simulink model "TV_2017old"  (R2016a)
settings: Solver=FixedStepAuto  StartTime=0.0  StopTime=inf  FixedStep=0.001  RelTol=1e-3
PreLoadFcn:
  | TV_2017_parameters
values from neighbouring files (symbols this model uses):
  battery_voltage = single(530)    [HIL_parameters.m]    (also in HIL_parameters_2018.m; TV_2017_parameters.m; TV_2017_parameters_VD.m)
  car_params = Simulink_Car_params    [HIL_parameters.m]    (also in HIL_parameters_2018.m; TV_2017_parameters.m; TV_2017_parameters_VD.m)
  i_Diff = 16    [HIL_parameters.m]    (also in HIL_parameters_2018.m; TV_2017_parameters.m)
  Kp = 1    [HIL_parameters.m]    (also in HIL_parameters_2018.m; TV_2017_parameters.m; TV_2017_parameters_VD.m)
  motor_data = struct    [HIL_parameters.m]    (also in HIL_parameters_2018.m; TV_2017_parameters.m)
  powerLimitControl = Simulink_el    [HIL_parameters.m]    (also in HIL_parameters_2018.m; TV_2017_parameters.m; TV_2017_parameters_VD.m)
  settings = Simulink_Settings    [HIL_parameters.m]    (also in HIL_parameters_2018.m; TV_2017_parameters.m; TV_2017_parameters_VD.m)
  SpdC_BCC = 0    [HIL_parameters.m]    (also in HIL_parameters_2018.m; TV_2017_parameters.m; TV_2017_parameters_VD.m)
  Speed_Neg_sat = -21    [HIL_parameters.m]    (also in HIL_parameters_2018.m; TV_2017_parameters.m; TV_2017_parameters_VD.m)
  Speed_Pos_sat = 21    [HIL_parameters.m]    (also in HIL_parameters_2018.m; TV_2017_parameters.m; TV_2017_parameters_VD.m)
  SteeringAngleFL = [-23.80 -22.65 -21.50 -20.34 -19.18 -18.03 -16.86 -15.70 -14.53 -13.35 -12.18 -10.99 -9.80 -8.61 -7.40 -6.19 -4.97 -3.75 -2.51 -1.26 0 1.27 2.56 3.85 5.17 6.50 7.84 9.21 10.59 12.00 13.42 14.88 16.36 17.87 19.41 20.99 22.61 24.26 25.97 27.73 29.54]    [CarSetupAnalysis2018.m]    (also in HIL_parameters_2018.m; TV_2017_parameters.m; TV_2017_parameters_VD.m = [-24.129 -22.950 -21.772 -20.593 -19.413 -18.232 -17.050 -15)
  SteeringAngleFR = [-29.54 -27.73 -25.97 -24.26 -22.61 -20.99 -19.41 -17.87 -16.36 -14.88 -13.42 -12.00 -10.59 -9.21 -7.84 -6.50 -5.17 -3.85 -2.56 -1.27 0 1.26 2.51 3.75 4.97 6.19 7.40 8.61 9.80 10.99 12.18 13.35 14.53 15.70 16.86 18.03 19.18 20.34 21.50 22.65 23.80]    [CarSetupAnalysis2018.m]    (also in HIL_parameters_2018.m; TV_2017_parameters.m; TV_2017_parameters_VD.m = [-29.3050 -27.5340 -25.8140 -24.1410 -22.5110 -20.9180 -19.3)
  SteeringWhAngle = [-105 -99.75 -94.5 -89.25 -84 -78.75 -73.5 -68.25 -63 -57.75 -52.5 -47.25 -42 -36.75 -31.5 -26.25 -21.0 -15.75 -10.5 -5.25 0.0 5.25 10.50 15.75 21.00 26.25 31.50 36.75 42.00 47.25 52.50 57.75  63.00 68.25 73.50 78.75 84.00 89.25 94.50 99.75 105.00]    [TV_2017_parameters_VD.m]
  Tn_n = 0    [HIL_parameters.m]    (also in HIL_parameters_2018.m; TV_2017_parameters.m; TV_2017_parameters_VD.m)
  tractionControl = Simulink_tc    [HIL_parameters.m]    (also in HIL_parameters_2018.m; IterativeTractionControlTuning.m; TV_2017_parameters.m; TV_2017_parameters_VD.m)
  yawRateControl = Simulink_yawRate    [HIL_parameters.m]    (also in HIL_parameters_2018.m; TV_2017_parameters.m; TV_2017_parameters_VD.m)
undefined symbols (not defined in the file or in its folder): DiscIntNeverNeededParam, magnitude, speedEstimation, TC_Decr_Gas, TC_Derivative, TC_Incr_Gas, TC_On, TC_Relay_Off, TC_Relay_On
libraries: CarMaker4SL x274, simulink_extras x45, simulink x37, dspfdesign x2
(part 3 of 14)

== system TV_2017old/CarMaker/Control_System /2016 adapted ==
  note: This needs more thought
  Mz_ref : Inport
  T_req : Inport  Port=2
  "States " : Inport  Port=3
  Bus Selector : BusSelector  OutputSignals=mmt_FL,mmt_FR,mmt_RL,mmt_RR
  Constant{1..4} (4 alike) : Constant  Value=int8(0)
  Inverter temperature limiter : MATLAB Function  TreatAsAtomicUnit=on
  MATLAB Function : MATLAB Function  Commented=on  TreatAsAtomicUnit=on
  Motor temperature limiter : MATLAB Function  TreatAsAtomicUnit=on
  Mux18 : Mux
  Mux2 : Mux
  Torque Allocation : Subsystem
  "max combined tire torque based on (Fz, SA,mu) " : MATLAB Function  TreatAsAtomicUnit=on
  "max long tire torque based on (FZ , mu)" : MATLAB Function  TreatAsAtomicUnit=on
  "max torque " : MATLAB Function  TreatAsAtomicUnit=on
  maxMotorTorque and kers based on available power : MATLAB Function  TreatAsAtomicUnit=on
  maxmotortoruq : Scope
  "Mz_allocated " : Outport
  Ti_lim : Outport  Port=2
  saturated_constraints : Outport  Port=3
  Max_motor_torque : Outport  Port=4
  active_constraints : Outport  Port=5
  wires:
  "States "/1 -> [states], Torque Allocation/2(states)
  Mz_ref/1 -> Torque Allocation/4(Mz_ref)
  Bus Selector/1 -> Mux18/1  "<mmt_FL>"
  Bus Selector/2 -> Mux18/2  "<mmt_FR>"
  Bus Selector/3 -> Mux18/3  "<mmt_RL>"
  Bus Selector/4 -> Mux18/4  "<mmt_RR>"
  T_req/1 -> Torque Allocation/1(T_req)
  Torque Allocation/1(Ti_lim) -> Ti_lim/1
  Mux18/1 -> maxmotortoruq/1
  [states] -> maxMotorTorque and kers based on available power/1(states)
  Inverter temperature limiter/1(maxMotorTorque) -> "max torque "/1(calc_pow_lim), "max torque "/2(inv_temp_lim)
  "max torque "/1(maxMotorTorque) -> Max_motor_torque/1, Bus Selector/1, [maxMotorTorque]
  "max torque "/2(active_constraints) -> active_constraints/1, [active_constraints]
  [states] -> Inverter temperature limiter/1(states)
  Motor temperature limiter/1(maxMotorTorque) -> "max torque "/3(mot_temp_lim)
  [states] -> Motor temperature limiter/1(states)
  "max long tire torque based on (FZ , mu)"/1(maxMotorTorque) -> "max torque "/5(SA_lim), "max torque "/4(mu_lim)
  [states] -> "max long tire torque based on (FZ , mu)"/1(states)
  "max combined tire torque based on (Fz, SA,mu) "/1(maxMotorTorque) -> ?
  [states] -> "max combined tire torque based on (Fz, SA,mu) "/1(states)
  maxMotorTorque and kers based on available power/1(maxMotorTorque) -> ?
  Mux2/1 -> saturated_constraints/1
  Constant1/1 -> Mux2/1  "<mmt_FL>"
  Constant2/1 -> Mux2/2  "<mmt_FR>"
  Constant3/1 -> Mux2/3  "<mmt_RL>"
  Constant4/1 -> Mux2/4  "<mmt_RR>"
  Torque Allocation/2(Mz_allocated) -> "Mz_allocated "/1
  [maxMotorTorque] -> Torque Allocation/3(maxMotorTorque)

== system TV_2017old/CarMaker/Control_System /Output Interface reduce slipratio ==
  Ti_lim : Inport
  MATLAB Function : MATLAB Function  TreatAsAtomicUnit=on
  "Ti_pos " : Outport
  Ti_neg : Outport  Port=2
  wi_setpoints : Outport  Port=3
  wires:
  MATLAB Function/2(Ti_neg) -> Ti_neg/1
  Ti_lim/1 -> MATLAB Function/1(Ti)
  MATLAB Function/1(Ti_pos) -> "Ti_pos "/1
  MATLAB Function/3(wi_setpoints) -> wi_setpoints/1

== system TV_2017old/CarMaker/Control_System /Power Limit Torque Reduction Controller  ==
  note: Hvis enable == 2, input 1 blir passet
      | Hvis Enable == {1,2}, input 3 blir passet
  Ti_lim : Inport
  states : Inport  Port=2
  Bus Creator1 : BusCreator  Inputs=4  OutDataTypeStr=Bus: Ti_lim  NonVirtualBus=on
      settings: InheritFromInputs=off
  Bus Creator2 : BusCreator  Inputs=4  OutDataTypeStr=Bus: Motor_Efficiencies  NonVirtualBus=on
      settings: InheritFromInputs=off
  Motorestimates : Subsystem
  "Old powerlimiting " : Subsystem  Commented=on
  Powerlimiting_Control_block : MATLAB Function  TreatAsAtomicUnit=on  SystemSampleTime=0.01
  Scope1 : Scope  NumInputPorts=2
  Scope2 : Scope  NumInputPorts=2
  Scope3 : Scope  NumInputPorts=4
  Scope4 : Scope
  Scope8 : Scope  NumInputPorts=5
  Switch : Switch  Threshold=2
  To Workspace : ToWorkspace  VariableName=Powertest  SaveFormat=Timeseries  SampleTime=-1
  extractPower1 : MATLAB Function  TreatAsAtomicUnit=on
  t_lim : Outport
  wires:
  states/1 -> Powerlimiting_Control_block/1(states), extractPower1/1(states), "Old powerlimiting "/2(states), Motorestimates/1(states)
  Powerlimiting_Control_block/3(RL) -> Scope8/3, Bus Creator1/3
  Powerlimiting_Control_block/2(FR) -> Scope8/2, Bus Creator1/2
  Powerlimiting_Control_block/1(FL) -> Scope8/1, Bus Creator1/1
  Powerlimiting_Control_block/4(RR) -> Bus Creator1/4, Scope8/4
  Ti_lim/1 -> "Old powerlimiting "/1(ti_lim), Motorestimates/2(Ti_lim), Powerlimiting_Control_block/3(Ti_lim)
  Motorestimates/1(Eff_FL) -> Scope2/2, Bus Creator2/1
  Motorestimates/2(Eff_FR) -> Bus Creator2/2
  Motorestimates/3(Eff_RL) -> Bus Creator2/3
  Motorestimates/4(Eff_RR) -> Bus Creator2/4
  Bus Creator2/1 -> Powerlimiting_Control_block/2(Motor_Efficiencies)
  extractPower1/1(power) -> To Workspace/1, Scope1/2
  Bus Creator1/1 -> t_lim/1
  Powerlimiting_Control_block/6(test1) -> Scope3/1
  Powerlimiting_Control_block/7(test2) -> Scope3/2
  Powerlimiting_Control_block/8(test3) -> Scope3/3
  Powerlimiting_Control_block/9(test4) -> Scope3/4
  Powerlimiting_Control_block/5(state) -> Scope4/1

== system TV_2017old/CarMaker/Control_System /Slip Rate Control  ==
  Ti_ref : Inport
  "States " : Inport  Port=2
  T_req : Inport  Port=3
  Bus Selector : BusSelector  OutputSignals=FL,FR,RL,RR
  Constant : Constant  Value=0
  Index Vector : MultiPortSwitch  DataPortOrder=Zero-based contiguous  Inputs=2  zeroidx=on
  Mux18 : Mux
  SMC Traction Control : Subsystem  Commented=on
  SUM : Subsystem
  Traction Controllers : Subsystem
  tcOutput : Scope
  Ti_lim : Outport
  T_sum_TC : Outport  Port=2
  wires:
  "States "/1 -> Traction Controllers/1(states)
  Ti_ref/1 -> Traction Controllers/2(Ti_ref), Index Vector/2
  Index Vector/1 -> Ti_lim/1
  Constant/1 -> Index Vector/1
  T_req/1 -> Traction Controllers/3(T_requested)
  Mux18/1 -> tcOutput/1
  Bus Selector/1 -> Mux18/1  "<FL>"
  Bus Selector/2 -> Mux18/2  "<FR>"
  Bus Selector/3 -> Mux18/3  "<RL>"
  Bus Selector/4 -> Mux18/4  "<RR>"
  Traction Controllers/1(Ti_SR) -> SUM/1(In1), Bus Selector/1, Index Vector/3
  SUM/1(Out1) -> T_sum_TC/1

== system TV_2017old/CarMaker/Control_System /TA 2017 ==
  Mz_ref : Inport
  T_req : Inport  Port=2
  "States " : Inport  Port=3
  Bus Selector1 : BusSelector  OutputSignals=mmt_FL,mmt_FR,mmt_RL,mmt_RR
  Bus Selector2 : BusSelector  OutputSignals=mmt_FL,mmt_FR,mmt_RL,mmt_RR
  Bus Selector6 : BusSelector  OutputSignals=FL,FR,RL,RR
  Friction Torque Limits : Scope
  From7 : From  Commented=on  GotoTag=states
  From9 : From  Commented=on  GotoTag=states
  Inverter temperature limiter : MATLAB Function  Commented=on  TreatAsAtomicUnit=on
  Motor temperature limiter : MATLAB Function  Commented=on  TreatAsAtomicUnit=on
  Mux{1..3,7} (4 alike) : Mux
  Mz : Scope
  "T_req_scope " : Scope
  Ti_Lim_TA1 : Scope  NumInputPorts=4
  Ti_max : Scope
  Torque lim Slip : Scope
  TorqueAllocation : MATLAB Function  TreatAsAtomicUnit=on
  TorqueLimFZ : Scope
  "max combined tire torque based on (Fz, SA,mu) " : MATLAB Function  TreatAsAtomicUnit=on
  "max combined tire torque based on (Fz, SA,mu) 1" : MATLAB Function  TreatAsAtomicUnit=on
  "max long tire torque based on (FZ , mu)" : MATLAB Function  TreatAsAtomicUnit=on
  "max torque " : MATLAB Function  TreatAsAtomicUnit=on
  required torque : Scope  NumInputPorts=4
  "Mz_error " : Outport
  Ti_lim : Outport  Port=2
  pow_red : Outport  Port=3
  max_motor_torque : Outport  Port=4
  active_constraints : Outport  Port=5
  overiterate 1 : Outport  Port=6
  wires:
  Mux1/1 -> Mz/1
  TorqueAllocation/4(Mz_allocated) -> required torque/4, Mux1/2  "Mz_all"
  TorqueAllocation/2(pow_red) -> pow_red/1, Ti_max/1
  Mz_ref/1 -> required torque/2, Mux1/3, TorqueAllocation/1(Mz_ref)  "Mz_ref"
  "States "/1 -> [states], TorqueAllocation/3(states)
  "max torque "/2(active_constraints) -> [active_constraints]
  From7/1 -> Inverter temperature limiter/1(states)
  From9/1 -> Motor temperature limiter/1(states)
  "max long tire torque based on (FZ , mu)"/1(maxMotorTorque) -> Bus Selector2/1, "max torque "/2(SA_lim), "max torque "/4(mot_temp_lim), "max torque "/3(inv_temp_lim), "max torque "/1(mu_lim)
  [states] -> "max long tire torque based on (FZ , mu)"/1(states)
  [states] -> "max combined tire torque based on (Fz, SA,mu) "/1(states)
  [maxMotorTorque] -> max_motor_torque/1
  [active_constraints] -> active_constraints/1
  "max torque "/1(maxMotorTorque) -> [maxMotorTorque]
  [maxMotorTorque] -> TorqueAllocation/4(maxMotorTorque)
  TorqueAllocation/3(Mz_error) -> required torque/3, Mux1/1, "Mz_error "/1  "Mz_error"
  "max torque "/3(friction_limits) -> Friction Torque Limits/1, [friction_torque_limits]
  [friction_torque_limits] -> TorqueAllocation/5(friction_limit_torques)
  TorqueAllocation/5(overiterate) -> overiterate 1/1
  "max combined tire torque based on (Fz, SA,mu) "/1(maxMotorTorque) -> Bus Selector1/1
  [states] -> "max combined tire torque based on (Fz, SA,mu) 1"/1(states)
  T_req/1 -> "T_req_scope "/1, Mux1/4, required torque/1, TorqueAllocation/2(T_req)
  Bus Selector6/1 -> Ti_Lim_TA1/1, Mux7/1  "<FL>"
  Bus Selector6/2 -> Ti_Lim_TA1/2, Mux7/2  "<FR>"
  Bus Selector6/3 -> Ti_Lim_TA1/3, Mux7/3  "<RL>"
  Bus Selector6/4 -> Ti_Lim_TA1/4, Mux7/4  "<RR>"
  TorqueAllocation/1(Ti_lim) -> Bus Selector6/1, Ti_lim/1
  Mux7/1 -> ?
  Bus Selector1/1 -> Mux2/1  "<mmt_FL>"
  Bus Selector1/2 -> Mux2/2  "<mmt_FR>"
  Bus Selector1/3 -> Mux2/3  "<mmt_RL>"
  Bus Selector1/4 -> Mux2/4  "<mmt_RR>"
  Mux2/1 -> Torque lim Slip/1
  Bus Selector2/1 -> Mux3/1  "<mmt_FL>"
  Bus Selector2/2 -> Mux3/2  "<mmt_FR>"
  Bus Selector2/3 -> Mux3/3  "<mmt_RL>"
  Bus Selector2/4 -> Mux3/4  "<mmt_RR>"
  Mux3/1 -> TorqueLimFZ/1

== system TV_2017old/CarMaker/Control_System /Torque allocation 2016 ==
  Mz_ref : Inport
  T_req : Inport  Port=2
  "States " : Inport  Port=3
  Bus Selector : BusSelector  OutputSignals=mmt_FL,mmt_FR,mmt_RL,mmt_RR
  MATLAB Function : MATLAB Function  TreatAsAtomicUnit=on
  Mux18 : Mux
  Torque Allocation : Subsystem
  maxmotortoruq : Scope
  Ti_lim : Outport
  "Mz_error " : Outport  Port=2
  Max_motor_torque_i : Outport  Port=3
  wires:
  "States "/1 -> MATLAB Function/1(states), Torque Allocation/2(states)
  Mz_ref/1 -> Torque Allocation/4(Mz_ref)
  Torque Allocation/2(Mz_error) -> "Mz_error "/1
  MATLAB Function/1(maxMotorTorque) -> Bus Selector/1, Torque Allocation/3(maxMotorTorque)
  Bus Selector/1 -> Mux18/1  "<mmt_FL>"
  Bus Selector/2 -> Mux18/2  "<mmt_FR>"
  Bus Selector/3 -> Mux18/3  "<mmt_RL>"
  Bus Selector/4 -> Mux18/4  "<mmt_RR>"
  T_req/1 -> Torque Allocation/1(T_req)
  Torque Allocation/1(Ti_lim) -> Ti_lim/1
  Mux18/1 -> Max_motor_torque_i/1, maxmotortoruq/1

== system TV_2017old/CarMaker/Control_System /Torque allocation 2017 ==
  Mz_ref : Inport
  T_req : Inport  Port=2
  "States " : Inport  Port=3
  Bus Creator : BusCreator  Commented=on  Inputs=2  OutDataTypeStr=Bus: maxMotorTorque
  Bus Selector1 : BusSelector  Commented=on  OutputSignals=mmt_FL,mmt_FR,mmt_RL,mmt_RR
  Constant{1..4} (4 alike) : Constant  Value=int8(1)
  Inverter temperature limiter : MATLAB Function  TreatAsAtomicUnit=on
  Motor temperature limiter : MATLAB Function  TreatAsAtomicUnit=on
  Mux2 : Mux
  Scope : Scope
  Scope1 : Scope  Commented=on  NumInputPorts=4
  Torque Allocation Quadratic Programming : MATLAB Function  TreatAsAtomicUnit=on
  "max combined tire torque based on (Fz, SA,mu) " : MATLAB Function  TreatAsAtomicUnit=on
  "max long tire torque based on (FZ , mu)" : MATLAB Function  TreatAsAtomicUnit=on
  "max torque " : MATLAB Function  TreatAsAtomicUnit=on
  maxMotorTorque and kers based on available power : MATLAB Function  TreatAsAtomicUnit=on
  "Mz_allocated " : Outport
  Ti_lim : Outport  Port=2
  saturated_constraints : Outport  Port=3
  max_motor_torque : Outport  Port=4
  active_constraints : Outport  Port=5
  wires:
  [states] -> maxMotorTorque and kers based on available power/1(states)
  "max torque "/2(active_constraints) -> [active_constraints]
  [states] -> Inverter temperature limiter/1(states)
  Motor temperature limiter/1(maxMotorTorque) -> "max torque "/4(mot_temp_lim)
  [states] -> Motor temperature limiter/1(states)
  "max long tire torque based on (FZ , mu)"/1(maxMotorTorque) -> "max torque "/2(SA_lim), "max torque "/1(mu_lim)
  [states] -> "max long tire torque based on (FZ , mu)"/1(states)
  [states] -> "max combined tire torque based on (Fz, SA,mu) "/1(states)
  [maxMotorTorque] -> max_motor_torque/1
  [active_constraints] -> active_constraints/1
  Mux2/1 -> saturated_constraints/1
  Constant1/1 -> Mux2/1  "<mmt_FL>"
  Constant2/1 -> Mux2/2  "<mmt_FR>"
  Constant3/1 -> Mux2/3  "<mmt_RL>"
  Constant4/1 -> Mux2/4  "<mmt_RR>"
  Mz_ref/1 -> ?  "Mz_ref"
  T_req/1 -> ?
  "States "/1 -> [states]
  [states] -> ?
  [maxMotorTorque] -> ?
  ? -> Ti_lim/1
  ? -> "Mz_allocated "/1
  "max torque "/1(maxMotorTorque) -> Bus Selector1/1, [maxMotorTorque]
  Bus Selector1/1 -> Scope1/1  "<mmt_FL>"
  Bus Selector1/2 -> Scope1/2  "<mmt_FR>"
  Bus Selector1/3 -> Scope1/3  "<mmt_RL>"
  Bus Selector1/4 -> Scope1/4  "<mmt_RR>"
  Inverter temperature limiter/1(maxMotorTorque) -> "max torque "/3(inv_temp_lim)
  "max combined tire torque based on (Fz, SA,mu) "/1(maxMotorTorque) -> ?

== system TV_2017old/CarMaker/Control_System /Torque allocation QP- ==
  Mz_ref : Inport
  T_req : Inport  Port=2
  "States " : Inport  Port=3
  Bus Creator : BusCreator  Commented=on  Inputs=2  OutDataTypeStr=Bus: maxMotorTorque
  Bus Selector1 : BusSelector  OutputSignals=mmt_FL,mmt_FR,mmt_RL,mmt_RR
  Constant{1..4} (4 alike) : Constant  Value=int8(1)
  Inverter temperature limiter : MATLAB Function  TreatAsAtomicUnit=on
  Motor temperature limiter : MATLAB Function  TreatAsAtomicUnit=on
  Mux2 : Mux
  Scope : Scope
  Scope1 : Scope  NumInputPorts=4
  Torque Allocation Quadratic Programming : MATLAB Function  TreatAsAtomicUnit=on
  "max combined tire torque based on (Fz, SA,mu) " : MATLAB Function  TreatAsAtomicUnit=on
  "max long tire torque based on (FZ , mu)" : MATLAB Function  TreatAsAtomicUnit=on
  "max torque " : MATLAB Function  TreatAsAtomicUnit=on
  maxMotorTorque and kers based on available power : MATLAB Function  TreatAsAtomicUnit=on
  "Mz_allocated " : Outport
  Ti_lim : Outport  Port=2
  saturated_constraints : Outport  Port=3
  max_motor_torque : Outport  Port=4
  active_constraints : Outport  Port=5
  wires:
  [states] -> maxMotorTorque and kers based on available power/1(states)
  "max torque "/2(active_constraints) -> [active_constraints]
  [states] -> Inverter temperature limiter/1(states)
  Motor temperature limiter/1(maxMotorTorque) -> "max torque "/4(mot_temp_lim)
  [states] -> Motor temperature limiter/1(states)
  "max long tire torque based on (FZ , mu)"/1(maxMotorTorque) -> "max torque "/2(SA_lim), "max torque "/1(mu_lim)
  [states] -> "max long tire torque based on (FZ , mu)"/1(states)
  [states] -> "max combined tire torque based on (Fz, SA,mu) "/1(states)
  [maxMotorTorque] -> max_motor_torque/1
  [active_constraints] -> active_constraints/1
  Mux2/1 -> saturated_constraints/1
  Constant1/1 -> Mux2/1  "<mmt_FL>"
  Constant2/1 -> Mux2/2  "<mmt_FR>"
  Constant3/1 -> Mux2/3  "<mmt_RL>"
  Constant4/1 -> Mux2/4  "<mmt_RR>"
  Mz_ref/1 -> Torque Allocation Quadratic Programming/1(Mz_ref)  "Mz_ref"
  T_req/1 -> Torque Allocation Quadratic Programming/2(T_req)
  "States "/1 -> [states]
  [states] -> Torque Allocation Quadratic Programming/3(states)
  [maxMotorTorque] -> Torque Allocation Quadratic Programming/4(maxMotorTorque)
  Torque Allocation Quadratic Programming/1(Ti_lim) -> Ti_lim/1
  Torque Allocation Quadratic Programming/3(Mz_allocated) -> "Mz_allocated "/1
  "max torque "/1(maxMotorTorque) -> Bus Selector1/1, [maxMotorTorque]
  Bus Selector1/1 -> Scope1/1  "<mmt_FL>"
  Bus Selector1/2 -> Scope1/2  "<mmt_FR>"
  Bus Selector1/3 -> Scope1/3  "<mmt_RL>"
  Bus Selector1/4 -> Scope1/4  "<mmt_RR>"
  Inverter temperature limiter/1(maxMotorTorque) -> "max torque "/3(inv_temp_lim)

== system TV_2017old/CarMaker/Control_System /Torque allocation QP-1 ==
  Mz_ref : Inport
  T_req : Inport  Port=2
  "States " : Inport  Port=3
  Bus Creator : BusCreator  Commented=on  Inputs=2  OutDataTypeStr=Bus: maxMotorTorque
  Bus Selector1 : BusSelector  OutputSignals=mmt_FL,mmt_FR,mmt_RL,mmt_RR
  Constant{1..4} (4 alike) : Constant  Value=int8(1)
  Inverter temperature limiter : MATLAB Function  TreatAsAtomicUnit=on
  Motor temperature limiter : MATLAB Function  TreatAsAtomicUnit=on
  Mux2 : Mux
  Scope : Scope
  Scope1 : Scope  NumInputPorts=4
  Torque Allocation Quadratic Programming : MATLAB Function  TreatAsAtomicUnit=on
  "max combined tire torque based on (Fz, SA,mu) " : MATLAB Function  TreatAsAtomicUnit=on
  "max long tire torque based on (FZ , mu)" : MATLAB Function  TreatAsAtomicUnit=on
  "max torque " : MATLAB Function  TreatAsAtomicUnit=on
  maxMotorTorque and kers based on available power : MATLAB Function  TreatAsAtomicUnit=on
  "Mz_allocated " : Outport
  Ti_lim : Outport  Port=2
  saturated_constraints : Outport  Port=3
  max_motor_torque : Outport  Port=4
  active_constraints : Outport  Port=5
  wires:
  [states] -> maxMotorTorque and kers based on available power/1(states)
  "max torque "/2(active_constraints) -> [active_constraints]
  [states] -> Inverter temperature limiter/1(states)
  Motor temperature limiter/1(maxMotorTorque) -> "max torque "/4(mot_temp_lim)
  [states] -> Motor temperature limiter/1(states)
  "max long tire torque based on (FZ , mu)"/1(maxMotorTorque) -> "max torque "/2(SA_lim), "max torque "/1(mu_lim)
  [states] -> "max long tire torque based on (FZ , mu)"/1(states)
  [states] -> "max combined tire torque based on (Fz, SA,mu) "/1(states)
  [maxMotorTorque] -> max_motor_torque/1
  [active_constraints] -> active_constraints/1
  Mux2/1 -> saturated_constraints/1
  Constant1/1 -> Mux2/1  "<mmt_FL>"
  Constant2/1 -> Mux2/2  "<mmt_FR>"
  Constant3/1 -> Mux2/3  "<mmt_RL>"
  Constant4/1 -> Mux2/4  "<mmt_RR>"
  Mz_ref/1 -> Torque Allocation Quadratic Programming/1(Mz_ref)  "Mz_ref"
  T_req/1 -> Torque Allocation Quadratic Programming/2(T_req)
  "States "/1 -> [states]
  [states] -> Torque Allocation Quadratic Programming/3(states)
  [maxMotorTorque] -> Torque Allocation Quadratic Programming/4(maxMotorTorque)
  Torque Allocation Quadratic Programming/1(Ti_lim) -> Ti_lim/1
  Torque Allocation Quadratic Programming/3(Mz_allocated) -> "Mz_allocated "/1
  "max torque "/1(maxMotorTorque) -> Bus Selector1/1, [maxMotorTorque]
  Bus Selector1/1 -> Scope1/1  "<mmt_FL>"
  Bus Selector1/2 -> Scope1/2  "<mmt_FR>"
  Bus Selector1/3 -> Scope1/3  "<mmt_RL>"
  Bus Selector1/4 -> Scope1/4  "<mmt_RR>"
  Inverter temperature limiter/1(maxMotorTorque) -> "max torque "/3(inv_temp_lim)

== system TV_2017old/CarMaker/Control_System /Yaw Rate Controller  ==
  "Mz_error " : Inport
  States : Inport  Port=2
  Data Type Conversion : DataTypeConversion  OutDataTypeStr=single  RndMeth=Round
  Discrete-Time Integrator2 : DiscreteIntegrator  InitialConditionSetting=State (most efficient)  SampleTime=-1  LimitOutput=on  UpperSaturationLimit=yawRateControl.max_moment  LowerSaturationLimit=-yawRateControl.max_moment  ICPrevOutput=DiscIntNeverNeededParam  ICPrevScaledInput=DiscIntNeverNeededParam
  Enable/disable : Constant  Value=yawRateControl.enable
  ErrorSerch_YRR : Scope  NumInputPorts=3
  Gain1 : Gain  Gain=single(3.6)
  Ksat : Constant  Value=yawRateControl.Ksat
  Memory : Memory  InheritSampleTime=on
  Mz_ref_YRR : Scope  NumInputPorts=2
  "Mzerror " : Scope
  Mzerror 1 : Scope  NumInputPorts=2
  PI_Ki 3 : Scope
  Product{7..8,10..11} (4 alike) : Product
  Product3 : Product  OutDataTypeStr=single
  Saturation : Saturate  UpperLimit=yawRateControl.max_moment  LowerLimit=-yawRateControl.max_moment
  Sum2 : Sum  Inputs=+++  AccumDataTypeStr=single
  Sum3 : Sum  Inputs=|+-
  gainScheduling : MATLAB Function  TreatAsAtomicUnit=on
  "not NaN " : MATLAB Function  TreatAsAtomicUnit=on
  not not a number : MATLAB Function  TreatAsAtomicUnit=on
  yawRateReference : MATLAB Function  TreatAsAtomicUnit=on
  "r_ref " : Outport
  r_lim : Outport  Port=2
  ay_max : Outport  Port=3
  Mz_ref : Outport  Port=4  OutDataTypeStr=single
  Mz_ref_to_telemetry : Outport  Port=5  OutDataTypeStr=single
  wires:
  States/1 -> yawRateReference/1(states)
  yawRateReference/4(r_ref) -> ErrorSerch_YRR/3, "r_ref "/1
  yawRateReference/5(r_lim) -> r_lim/1
  yawRateReference/6(ay_max) -> ay_max/1
  Product7/1 -> Sum2/2
  Sum2/1 -> Mz_ref_to_telemetry/1, Product3/2
  Product8/1 -> Sum3/1
  Sum3/1 -> Discrete-Time Integrator2/1
  Discrete-Time Integrator2/1 -> PI_Ki 3/1, Sum2/3
  Product11/1 -> not not a number/1(in)
  yawRateReference/1(r_der_error) -> Product10/1
  Product10/1 -> Sum2/1
  gainScheduling/2(Kp) -> Mzerror 1/1, Product7/1
  Ksat/1 -> Product11/1
  "Mz_error "/1 -> "Mzerror "/1, Product11/2
  gainScheduling/3(Ki) -> Product8/1, Mzerror 1/2
  yawRateReference/2(r_error) -> Memory/1, ErrorSerch_YRR/1, Product8/2, Product7/2
  Product3/1 -> Saturation/1
  Enable/disable/1 -> Product3/1
  yawRateReference/3(vx) -> Gain1/1
  Gain1/1 -> gainScheduling/1(vx_kmh)
  gainScheduling/1(Kd) -> Product10/2
  not not a number/1(out) -> Sum3/2
  Saturation/1 -> "not NaN "/1(in)
  "not NaN "/1(out) -> Data Type Conversion/1, Mz_ref_YRR/1
  Data Type Conversion/1 -> Mz_ref_YRR/2, Mz_ref/1
  Memory/1 -> yawRateReference/2(prev_r_error)

== system TV_2017old/CarMaker/Debug Information /Extract and scale to deg compare to CM output in individual error ==
  SA_CM : Inport
  In1 : Inport  Port=2
  Bus Selector1 : BusSelector  OutputSignals=FL,FR,RL,RR
  Demux : Demux
  Rate Transition2 : RateTransition  OutPortSampleTime=0.001
  SA  estimate : Scope  NumInputPorts=4
  Sum{,1..3} (4 alike) : Sum  Inputs=|-+
  r2d{,1..3} (4 alike) : simulink_extras/Transformations/Radians to Degrees
  FL : Outport
  FR : Outport  Port=2
  RL : Outport  Port=3
  RR : Outport  Port=4
  wires:
  SA_CM/1 -> Demux/1
  Demux/1 -> Sum/1
  r2d/1 -> Sum/2, SA  estimate/1
  Demux/2 -> Sum1/1
  r2d1/1 -> Sum1/2, SA  estimate/2
  Demux/3 -> Sum2/1
  r2d2/1 -> Sum2/2, SA  estimate/3
  Demux/4 -> Sum3/1
  r2d3/1 -> SA  estimate/4, Sum3/2
  Sum/1 -> FL/1
  Sum1/1 -> FR/1
  Sum2/1 -> RL/1
  Sum3/1 -> RR/1
  In1/1 -> Rate Transition2/1
  Bus Selector1/1 -> r2d/1  "<FL>"
  Bus Selector1/2 -> r2d1/1  "<FR>"
  Bus Selector1/3 -> r2d2/1  "<RL>"
  Bus Selector1/4 -> r2d3/1  "<RR>"
  Rate Transition2/1 -> Bus Selector1/1

== system TV_2017old/CarMaker/Debug Information /Extract and scale to deg compare to CM output in individual error1 ==
  SA_CM : Inport
  In1 : Inport  Port=2
  Bus Selector1 : BusSelector  OutputSignals=SR_FL,SR_FR,SR_RL,SR_RR
  Demux : Demux
  Rate Transition2 : RateTransition  OutPortSampleTime=0.001
  SR  estimate : Scope  NumInputPorts=4
  Sum{,1..3} (4 alike) : Sum  Inputs=|-+
  r2d{,1..3} (4 alike) : simulink_extras/Transformations/Radians to Degrees  Commented=on
  FL : Outport
  FR : Outport  Port=2
  RL : Outport  Port=3
  RR : Outport  Port=4
  wires:
  SA_CM/1 -> Demux/1
  Demux/1 -> Sum/1
  Demux/2 -> Sum1/1
  Demux/3 -> Sum2/1
  Demux/4 -> Sum3/1
  Sum/1 -> FL/1
  Sum1/1 -> FR/1
  Sum2/1 -> RL/1
  Sum3/1 -> RR/1
  In1/1 -> Rate Transition2/1
  Bus Selector1/1 -> Sum/2, SR  estimate/1  "<SR_FL>"
  Bus Selector1/2 -> Sum1/2, SR  estimate/2  "<SR_FR>"
  Bus Selector1/3 -> Sum2/2, SR  estimate/3  "<SR_RL>"
  Bus Selector1/4 -> SR  estimate/4, Sum3/2  "<SR_RR>"
  Rate Transition2/1 -> Bus Selector1/1

== system TV_2017old/CarMaker/Debug Information /Fz_Estimation ==
  sensors : Inport
  v_x : Inport  Port=2
  Bus Selector : BusSelector  OutputSignals=damper_rate_FL,damper_rate_FR,damper_rate_RL,damper_rate_RR
  Bus Selector1 : BusSelector  OutputSignals=FL,FR,RL,RR
  Bus Selector2 : BusSelector  OutputSignals=FL,FR,RL,RR
  Constant : Constant  Value=settings.select_Fz_est_method
  DamperRateLookup : Lookup_n-D  NumberOfTableDimensions=1  BreakpointsForDimension1=car_params.damper_table_breakpoint;  Table=car_params.damper_pull_push_values_front;  ExtrapMethod=Clip  UseLastTableValue=on  InternalRulePriority=Speed  RndMeth=Simplest  InputSameDT=on
  DamperRateLookup1 : Lookup_n-D  NumberOfTableDimensions=1  BreakpointsForDimension1=car_params.damper_table_breakpoint;  Table=car_params.damper_pull_push_values_front;  ExtrapMethod=Clip  UseLastTableValue=on  InternalRulePriority=Speed  RndMeth=Simplest  InputSameDT=on
  DamperRateLookup2 : Lookup_n-D  NumberOfTableDimensions=1  BreakpointsForDimension1=car_params.damper_table_breakpoint;  Table=car_params.damper_pull_push_values_rear;  ExtrapMethod=Clip  UseLastTableValue=on  InternalRulePriority=Speed  RndMeth=Simplest  InputSameDT=on
  DamperRateLookup3 : Lookup_n-D  NumberOfTableDimensions=1  BreakpointsForDimension1=car_params.damper_table_breakpoint;  Table=car_params.damper_pull_push_values_rear;  ExtrapMethod=Clip  UseLastTableValue=on  InternalRulePriority=Speed  RndMeth=Simplest  InputSameDT=on
  DamperRateLookup4 : Lookup_n-D  Commented=on  NumberOfTableDimensions=1  BreakpointsForDimension1=single([-200,0,200]);  Table=single([-500,0,500]);  ExtrapMethod=Clip  UseLastTableValue=on  InternalRulePriority=Speed  RndMeth=Simplest  InputSameDT=on
  DamperRateLookup5 : Lookup_n-D  Commented=on  NumberOfTableDimensions=1  BreakpointsForDimension1=single([-200,0,200]);  Table=single([-500,0,500]);  ExtrapMethod=Clip  UseLastTableValue=on  InternalRulePriority=Speed  RndMeth=Simplest  InputSameDT=on
  FzEstDamper : MATLAB Function  TreatAsAtomicUnit=on
  FzEstDamper 2016 : MATLAB Function  Commented=on  TreatAsAtomicUnit=on
  FzEstLoadTransfer : MATLAB Function  TreatAsAtomicUnit=on
  Index Vector : MultiPortSwitch  Inputs=2
  Scope : Scope  NumInputPorts=4
  Scope1 : Scope  NumInputPorts=4
  Fz_est : Outport
  Fz_LoadTransfer_est : Outport  Port=2
  Fz_damper_est : Outport  Port=3
  alfa_r : Outport  Port=4
  wires:
  sensors/1 -> FzEstLoadTransfer/1(sensor), FzEstDamper/1(sensors), Bus Selector/1
  DamperRateLookup/1 -> FzEstDamper/2(Fz_damp_FL)  "Fz_damp_FL"
  Bus Selector/1 -> DamperRateLookup/1  "<damper_rate_FL>"
  Bus Selector/2 -> DamperRateLookup1/1  "<damper_rate_FR>"
  Bus Selector/3 -> DamperRateLookup2/1  "<damper_rate_RL>"
  Bus Selector/4 -> DamperRateLookup3/1  "<damper_rate_RR>"
  DamperRateLookup1/1 -> FzEstDamper/3(Fz_damp_FR)
  DamperRateLookup2/1 -> FzEstDamper/4(Fz_damp_RL)
  DamperRateLookup3/1 -> FzEstDamper/5(Fz_damp_RR)
  Index Vector/1 -> Fz_est/1
  v_x/1 -> FzEstLoadTransfer/2(vx)
  FzEstDamper/2(alfa_r) -> alfa_r/1
  Bus Selector1/2 -> Scope/2  "<FR>"
  Bus Selector1/1 -> Scope/1  "<FL>"
  Bus Selector1/3 -> Scope/3  "<RL>"
  Bus Selector1/4 -> Scope/4  "<RR>"
  Constant/1 -> Index Vector/1
  FzEstLoadTransfer/1(Fz_loadTransfer_est) -> Bus Selector2/1, Fz_LoadTransfer_est/1, Index Vector/2
  Bus Selector2/2 -> Scope1/2  "<FR>"
  Bus Selector2/1 -> Scope1/1  "<FL>"
  Bus Selector2/3 -> Scope1/3  "<RL>"
  Bus Selector2/4 -> Scope1/4  "<RR>"
  FzEstDamper/1(Fz_damper_est) -> Index Vector/3, Bus Selector1/1, Fz_damper_est/1
  DamperRateLookup4/1 -> FzEstDamper 2016/3(Fz_damp_FR)
  DamperRateLookup5/1 -> FzEstDamper 2016/4(Fz_damp_RL)

== system TV_2017old/CarMaker/Debug Information /Mechanical effect ==
  Gain{8,16..17,19} (4 alike) : Gain  Gain=1/car_params.GR
  Gain{18,20..22} (4 alike) : Gain  Gain=car_params.GR
  Mux7 : Mux
  Pmechanical : Scope
  Product{,1..3} (4 alike) : Product
  Read CM Dict12 : CarMaker4SL/Read CM Dict  xname=Car.WheelSpd_RL  xsync=off
  Read CM Dict13 : CarMaker4SL/Read CM Dict  xname=Car.WheelSpd_FR  xsync=off
  Read CM Dict14 : CarMaker4SL/Read CM Dict  xname=Car.WheelSpd_FL  xsync=off
  Read CM Dict15 : CarMaker4SL/Read CM Dict  xname=PT.WFL.Trq_Drive  xsync=off
  Read CM Dict16 : CarMaker4SL/Read CM Dict  xname=Car.WheelSpd_RR  xsync=off
  Read CM Dict45 : CarMaker4SL/Read CM Dict  xname=PT.WFR.Trq_Drive  xsync=off
  Read CM Dict46 : CarMaker4SL/Read CM Dict  xname=PT.WRL.Trq_Drive  xsync=off
  Read CM Dict47 : CarMaker4SL/Read CM Dict  xname=PT.WRR.Trq_Drive  xsync=off
  To File10 : ToFile  Filename=MAT_files\MechanicalEffect.mat  MatrixName=MechEffect  SaveFormat=Timeseries
  wires:
  Mux7/1 -> Pmechanical/1, To File10/1
  Read CM Dict12/1 -> Gain18/1
  Gain17/1 -> Product1/1
  Read CM Dict14/1 -> Gain22/1
  Gain16/1 -> Product2/1
  Read CM Dict16/1 -> Gain20/1
  Gain19/1 -> Product/1
  Read CM Dict15/1 -> Gain16/1
  Read CM Dict45/1 -> Gain17/1
  Gain8/1 -> Product3/1
  Product1/1 -> Mux7/2  "FR"
  Product/1 -> Mux7/3  "RL"
  Gain22/1 -> Product2/2
  Gain21/1 -> Product1/2
  Read CM Dict47/1 -> Gain8/1
  Product3/1 -> Mux7/4  "RR"
  Read CM Dict13/1 -> Gain21/1
  Gain18/1 -> Product/2
  Gain20/1 -> Product3/2
  Read CM Dict46/1 -> Gain19/1
  Product2/1 -> Mux7/1  "FL"

== system TV_2017old/CarMaker/Debug Information /SA calculation ==
  In1 : Inport
  Bus Selector2 : BusSelector  OutputSignals=steering_wheel_angle
  Degrees to Radians : simulink_extras/Transformations/Degrees to Radians
  Degrees to Radians1 : simulink_extras/Transformations/Degrees to Radians
  FL steer ang lookup deg : Lookup_n-D  NumberOfTableDimensions=1  BreakpointsForDimension1=SteeringWhAngle  Table=SteeringAngleFL  ExtrapMethod=Clip  UseLastTableValue=on  InternalRulePriority=Speed  RndMeth=Simplest  InputSameDT=on
  FR steer ang lookup deg : Lookup_n-D  NumberOfTableDimensions=1  BreakpointsForDimension1=SteeringWhAngle  Table=SteeringAngleFR  ExtrapMethod=Clip  UseLastTableValue=on  InternalRulePriority=Speed  RndMeth=Simplest  InputSameDT=on
  Radians to Degrees1 : simulink_extras/Transformations/Radians to Degrees
  Slip angle calc : MATLAB Function  TreatAsAtomicUnit=on
  Out1 : Outport
  wires:
  Radians to Degrees1/1 -> FL steer ang lookup deg/1, FR steer ang lookup deg/1
  Degrees to Radians1/1 -> Slip angle calc/2(wheel_ang_right)
  Slip angle calc/1(SA) -> Out1/1
  FR steer ang lookup deg/1 -> Degrees to Radians1/1
  Degrees to Radians/1 -> Slip angle calc/1(wheel_ang_left)
  In1/1 -> Slip angle calc/3(sensor), Bus Selector2/1
  FL steer ang lookup deg/1 -> Degrees to Radians/1
  Bus Selector2/1 -> Radians to Degrees1/1  "<steering_wheel_angle>"

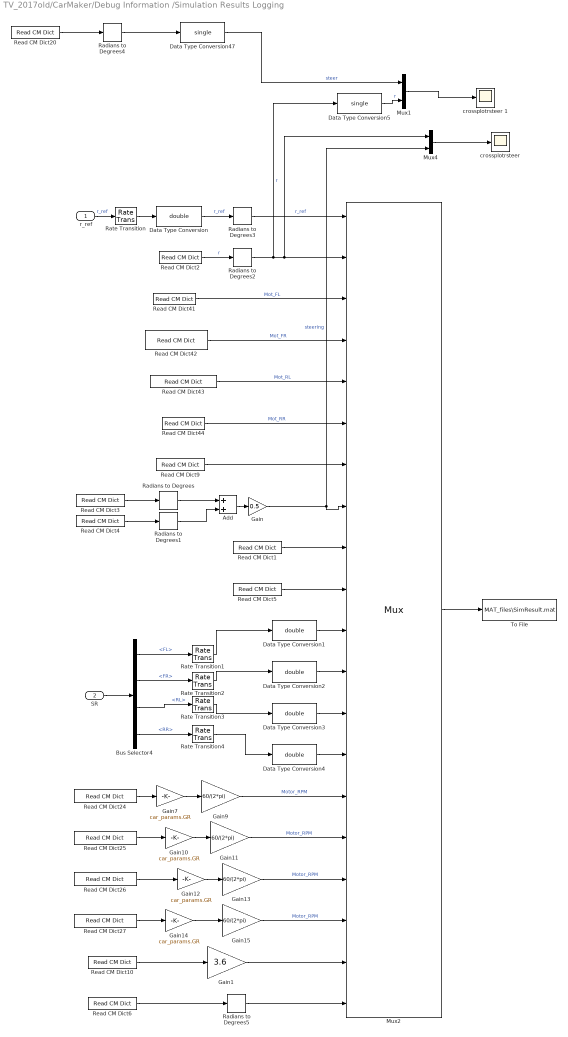
== system TV_2017old/CarMaker/Debug Information /Simulation Results Logging ==
  r_ref : Inport
  SR : Inport  Port=2
  Add : Sum
  Bus Selector4 : BusSelector  OutputSignals=FL,FR,RL,RR
  Data Type Conversion{,1..4} (5 alike) : DataTypeConversion  OutDataTypeStr=double
  Data Type Conversion47 : DataTypeConversion  OutDataTypeStr=single
  Data Type Conversion5 : DataTypeConversion  OutDataTypeStr=single
  Gain : Gain  Gain=0.5
  Gain1 : Gain  Gain=3.6
  Gain{7,10,12,14} (4 alike) : Gain  Gain=car_params.GR
  Gain{9,11,13,15} (4 alike) : Gain  Gain=60/(2*pi)
  Mux1 : Mux  Inputs=2
  Mux2 : Mux  Inputs=20
  Mux4 : Mux  Inputs=2
  Radians to Degrees{,1..5} (6 alike) : simulink_extras/Transformations/Radians to Degrees
  Rate Transition{,1..4} (5 alike) : RateTransition  OutPortSampleTime=0.001
  Read CM Dict1 : CarMaker4SL/Read CM Dict  xname=Vhcl.Fr1.x  xsync=off
  Read CM Dict10 : CarMaker4SL/Read CM Dict  xname=Car.vx  xsync=off
  Read CM Dict2 : CarMaker4SL/Read CM Dict  xname=Car.YawRate  xsync=off
  Read CM Dict20 : CarMaker4SL/Read CM Dict  xname=Vhcl.Steer.Ang  xsync=off
  Read CM Dict24 : CarMaker4SL/Read CM Dict  xname=Car.WheelSpd_FL  xsync=off
  Read CM Dict25 : CarMaker4SL/Read CM Dict  xname=Car.WheelSpd_FR  xsync=off
  Read CM Dict26 : CarMaker4SL/Read CM Dict  xname=Car.WheelSpd_RL  xsync=off
  Read CM Dict27 : CarMaker4SL/Read CM Dict  xname=Car.WheelSpd_RR  xsync=off
  Read CM Dict3 : CarMaker4SL/Read CM Dict  xname=Car.CFR.rz  xsync=off
  Read CM Dict4 : CarMaker4SL/Read CM Dict  xname=Car.CFL.rz  xsync=off
  Read CM Dict41 : CarMaker4SL/Read CM Dict  xname=PT.WFL.Trq_Drive  xsync=off
  Read CM Dict42 : CarMaker4SL/Read CM Dict  xname=PT.WFR.Trq_Drive  xsync=off
  Read CM Dict43 : CarMaker4SL/Read CM Dict  xname=PT.WRL.Trq_Drive  xsync=off
  Read CM Dict44 : CarMaker4SL/Read CM Dict  xname=PT.WRR.Trq_Drive  xsync=off
  Read CM Dict5 : CarMaker4SL/Read CM Dict  xname=Vhcl.Fr1.y  xsync=off
  Read CM Dict6 : CarMaker4SL/Read CM Dict  xname=Vhcl.Steer.Ang  xsync=off
  Read CM Dict9 : CarMaker4SL/Read CM Dict  xname=Car.ay  xsync=off
  To File : ToFile  Filename=MAT_files\SimResult.mat  MatrixName=sim  SaveFormat=Timeseries
  "crossplotrsteer " : Scope
  crossplotrsteer 1 : Scope
  wires:
  r_ref/1 -> Rate Transition/1  "r_ref"
  Read CM Dict2/1 -> Radians to Degrees2/1  "r"
  Data Type Conversion/1 -> Radians to Degrees3/1  "r_ref"
  Read CM Dict42/1 -> Mux2/4  "Mot_FR"
  Read CM Dict43/1 -> Mux2/5  "Mot_RL"
  Read CM Dict41/1 -> Mux2/3  "Mot_FL"
  Read CM Dict44/1 -> Mux2/6  "Mot_RR"
  Read CM Dict9/1 -> Mux2/7
  Read CM Dict3/1 -> Radians to Degrees/1
  Read CM Dict4/1 -> Radians to Degrees1/1
  Radians to Degrees/1 -> Add/1
  Radians to Degrees1/1 -> Add/2
  Radians to Degrees2/1 -> Data Type Conversion5/1, Mux4/1, Mux2/2  "r"
  Radians to Degrees3/1 -> Mux2/1  "r_ref"
  Add/1 -> Gain/1
  Mux2/1 -> To File/1
  Read CM Dict1/1 -> Mux2/9
  Read CM Dict5/1 -> Mux2/10
  Rate Transition/1 -> Data Type Conversion/1
  Mux4/1 -> "crossplotrsteer "/1
  Gain/1 -> Mux2/8, Mux4/2  "steering"
  Bus Selector4/1 -> Rate Transition1/1  "<FL>"
  Bus Selector4/2 -> Rate Transition2/1  "<FR>"
  Bus Selector4/3 -> Rate Transition3/1  "<RL>"
  Bus Selector4/4 -> Rate Transition4/1  "<RR>"
  SR/1 -> Bus Selector4/1
  Rate Transition1/1 -> Data Type Conversion1/1
  Rate Transition2/1 -> Data Type Conversion2/1
  Rate Transition3/1 -> Data Type Conversion3/1
  Rate Transition4/1 -> Data Type Conversion4/1
  Data Type Conversion1/1 -> Mux2/11
  Data Type Conversion2/1 -> Mux2/12
  Data Type Conversion3/1 -> Mux2/13
  Data Type Conversion4/1 -> Mux2/14
  Gain7/1 -> Gain9/1
  Gain9/1 -> Mux2/15  "Motor_RPM"
  Read CM Dict24/1 -> Gain7/1
  Read CM Dict25/1 -> Gain10/1
  Gain10/1 -> Gain11/1
  Gain11/1 -> Mux2/16  "Motor_RPM"
  Gain12/1 -> Gain13/1
  Gain13/1 -> Mux2/17  "Motor_RPM"
  Gain14/1 -> Gain15/1
  Gain15/1 -> Mux2/18  "Motor_RPM"
  Read CM Dict26/1 -> Gain12/1
  Read CM Dict27/1 -> Gain14/1
  Read CM Dict10/1 -> Gain1/1
  Gain1/1 -> Mux2/19
  Read CM Dict20/1 -> Radians to Degrees4/1
  Data Type Conversion47/1 -> Mux1/1  "steer"
  Mux1/1 -> crossplotrsteer 1/1
  Radians to Degrees4/1 -> Data Type Conversion47/1
  Data Type Conversion5/1 -> Mux1/2  "r"
  Read CM Dict6/1 -> Radians to Degrees5/1
  Radians to Degrees5/1 -> Mux2/20
